simulink model "System_noSolution"  (R2023a)
settings: Solver=VariableStepAuto  StartTime=0.0  StopTime=10.0  RelTol=1e-3
values from neighbouring files (symbols this model uses):
  A = ((2e-2)^2)*pi/4    (= 0.000314159265359)    [GeneralParameters_PID_LQR.m]
  n_cal = n_layers*turns_per_layer    (= 5412)    [GeneralParameters_PID_LQR.m]
  R_mgt = 30    [GeneralParameters_PID_LQR.m]
settings Model: Creator=Personal  LastModifiedBy=Personal

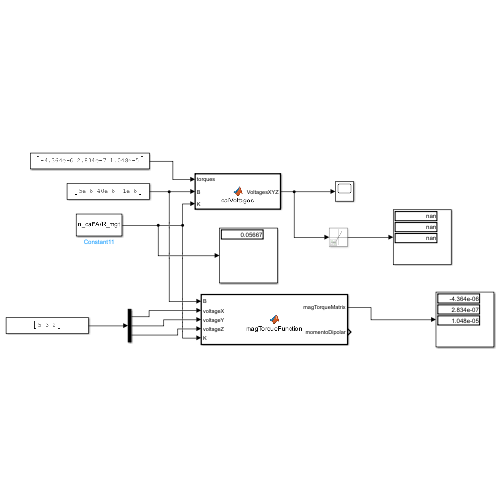
[thumbnail: Simulink's stored preview of the top-level diagram]
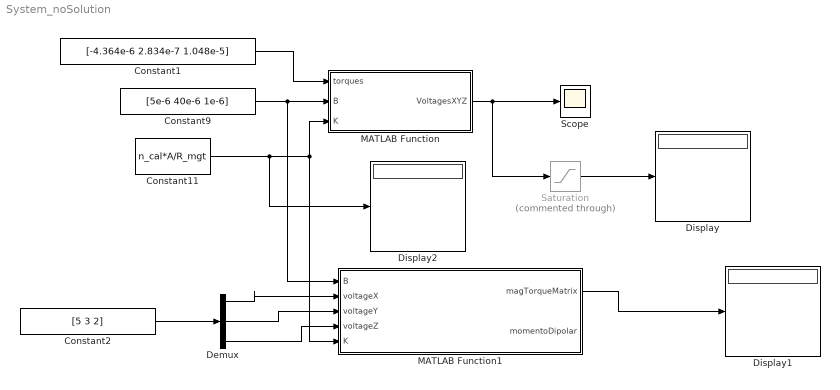
== system System_noSolution ==
  Constant1 : Constant  Value=[-4.364e-6 2.834e-7 1.048e-5]
  Constant11 : Constant  Value=n_cal*A/R_mgt
  Constant2 : Constant  Value=[5 3 2]
  Constant9 : Constant  Value=[5e-6 40e-6 1e-6]
  Demux : Demux  Outputs=3
  Display : Display
  Display1 : Display
  Display2 : Display
  MATLAB Function : MATLAB Function  TreatAsAtomicUnit=on
  MATLAB Function1 : MATLAB Function  TreatAsAtomicUnit=on
  Saturation : Saturate  Commented=through  UpperLimit=5  LowerLimit=-5
  Scope : Scope
  wires:
  Constant11/1 -> Display2/1, MATLAB Function1/5(K), MATLAB Function/3(K)
  Constant9/1 -> MATLAB Function1/1(B), MATLAB Function/2(B)
  Constant1/1 -> MATLAB Function/1(torques)
  MATLAB Function/1(VoltagesXYZ) -> Saturation/1, Scope/1
  Saturation/1 -> Display/1
  Demux/1 -> MATLAB Function1/2(voltageX)
  Demux/2 -> MATLAB Function1/3(voltageY)
  Demux/3 -> MATLAB Function1/4(voltageZ)
  Constant2/1 -> Demux/1
  MATLAB Function1/1(magTorqueMatrix) -> Display1/1

== matlab function System_noSolution/MATLAB Function1 ==
  data: B input; magTorqueMatrix output; voltageX input; voltageY input; voltageZ input; momentoDipolar output; K input
function [magTorqueMatrix,momentoDipolar] = magTorqueFunction(B,voltageX,voltageY,voltageZ,K)

%d = 1.45e-2; % Diametro mgt [m]
d = 1.45e-2; % Diametro mgt [m]
A =((2e-2)^2)*pi/4; % m^2

%n=sqrt(L*l/(mu_0*mu_r*A)); % # Vueltas 
n = 5412;

%R = 50.7 ;% Resistencia mgt [Ohm];
R = 30 ;% Resistencia mgt [Ohm];
ix = voltageX/R;
iy = voltageY/R;
iz = voltageZ/R;

% M = [n*ix*A n*iy*A n*iz*A]';
% 
% magTorqueMatrix = -skew(B)*M;

magTorqueMatrix_X = cross(voltageX*K*[1 0 0],B);
magTorqueMatrix_Y = cross(voltageY*K*[0 1 0],B);
magTorqueMatrix_Z = cross(voltageZ*K*[0 0 1],B);
 momentoDipolar = [n*ix*A n*iy*A n*iz*A];

magTorqueMatrix = magTorqueMatrix_X+magTorqueMatrix_Y+magTorqueMatrix_Z;

== matlab function System_noSolution/MATLAB Function ==
  data: torques input; VoltagesXYZ output; B input; K input
function VoltagesXYZ = calVoltages(torques,B,K)
Bx = B(1);
By = B(2);
Bz = B(3);

Tx = torques(1);
Ty = torques(2);
Tz = torques(3);


% syms Vx Vy Vz
% eqn1 = 0*Vx + K*Bz*Vy -K*By*Vz == Tx;
% eqn2 = -K*Bz*Vx + 0*Vy +K*Bx*Vz == Ty;
% eqn3 = K*By*Vx -K*Bx*Vy +0*Vz == Tz;
% 
% [A,B] = equationsToMatrix([eqn1, eqn2, eqn3], [Vx, Vy, Vz]);

A = [0 K*Bz -K*By;
    -K*Bz 0 K*Bx;
    K*By -K*Bx 0];
B = torques;

VoltagesXYZ = A^-1*B;
end
